simulink model "hw1_simu"  (R2015a)
settings: Solver=ode4  StartTime=0.0  StopTime=20.0  FixedStep=0.0278  RelTol=1e-3
settings Model: Creator=DELL-  LastModifiedBy=DELL-

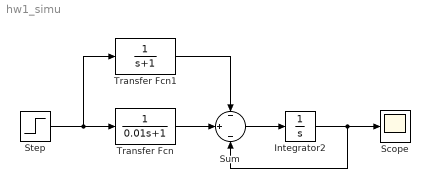
== system hw1_simu ==
  Integrator2 : Integrator
  Scope : Scope
  Step : Step  Time=0  SampleTime=0
  Sum : Sum  Inputs=-|+|-
  Transfer Fcn : TransferFcn  Denominator=[0.01 1]
  Transfer Fcn1 : TransferFcn  Denominator=[1 1]
  wires:
  Step/1 -> Transfer Fcn1/1, Transfer Fcn/1
  Integrator2/1 -> Sum/3, Scope/1
  Transfer Fcn1/1 -> Sum/1
  Sum/1 -> Integrator2/1
  Transfer Fcn/1 -> Sum/2
